simulink model "Lab5"  (R2017b)
settings: Solver=VariableStepAuto  StartTime=0.0  StopTime=200  RelTol=1e-3
libraries: cstblocks x8
settings Model: Creator=kelem  LastModifiedBy=kelem

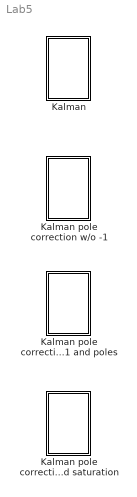
== system Lab5 ==
  Kalman : Subsystem
  Kalman pole correction w/o -1 : Subsystem
  Kalman pole correction1 w/o -1 and poles : Subsystem
  Kalman pole correction1 w/o -1 and poles and saturation : Subsystem

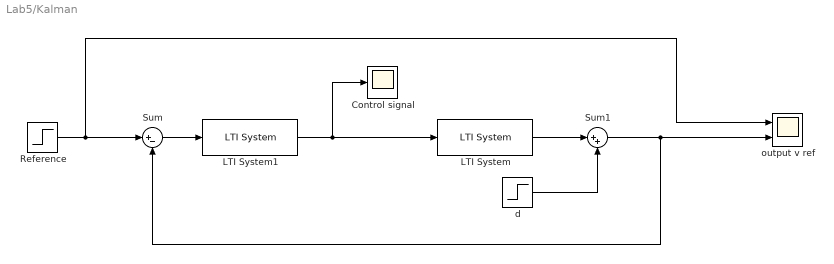
== system Lab5/Kalman ==
  "Control signal " : Scope
  LTI System : cstblocks/LTI System  sys=Hf  IC=[]
  LTI System1 : cstblocks/LTI System  sys=Hkc1  IC=[]
  Reference : Step  SampleTime=0
  Sum : Sum  Inputs=|+-
  Sum1 : Sum  Inputs=|++
  d : Step  SampleTime=50
  "output v ref " : Scope  NumInputPorts=2
  wires:
  LTI System1/1 -> LTI System/1, "Control signal "/1
  Sum/1 -> LTI System1/1
  d/1 -> Sum1/2
  Reference/1 -> Sum/1, "output v ref "/1
  Sum1/1 -> Sum/2, "output v ref "/2
  LTI System/1 -> Sum1/1

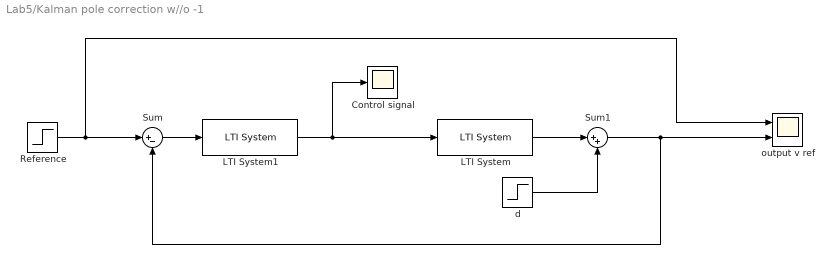
== system Lab5/Kalman pole correction w//o -1 ==
  "Control signal " : Scope
  LTI System : cstblocks/LTI System  sys=Hf  IC=[]
  LTI System1 : cstblocks/LTI System  sys=Hkc2  IC=[]
  Reference : Step  SampleTime=0
  Sum : Sum  Inputs=|+-
  Sum1 : Sum  Inputs=|++
  d : Step  SampleTime=50
  "output v ref " : Scope  NumInputPorts=2
  wires:
  LTI System1/1 -> LTI System/1, "Control signal "/1
  Sum/1 -> LTI System1/1
  d/1 -> Sum1/2
  Reference/1 -> Sum/1, "output v ref "/1
  Sum1/1 -> Sum/2, "output v ref "/2
  LTI System/1 -> Sum1/1

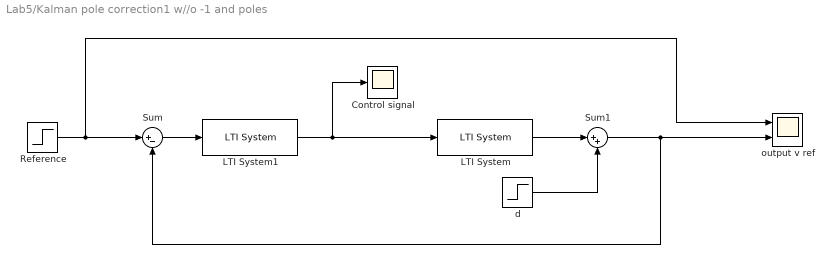
== system Lab5/Kalman pole correction1 w//o -1 and poles ==
  "Control signal " : Scope
  LTI System : cstblocks/LTI System  sys=Hf  IC=[]
  LTI System1 : cstblocks/LTI System  sys=Hkc3  IC=[]
  Reference : Step  SampleTime=0
  Sum : Sum  Inputs=|+-
  Sum1 : Sum  Inputs=|++
  d : Step  SampleTime=50
  "output v ref " : Scope  NumInputPorts=2
  wires:
  LTI System1/1 -> LTI System/1, "Control signal "/1
  Sum/1 -> LTI System1/1
  d/1 -> Sum1/2
  Reference/1 -> Sum/1, "output v ref "/1
  Sum1/1 -> Sum/2, "output v ref "/2
  LTI System/1 -> Sum1/1

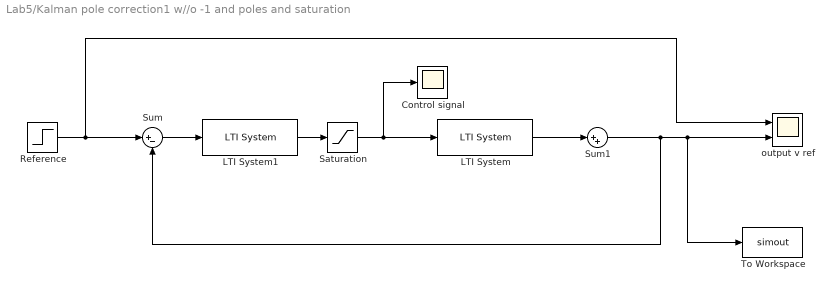
== system Lab5/Kalman pole correction1 w//o -1 and poles and saturation ==
  "Control signal " : Scope
  LTI System : cstblocks/LTI System  sys=Hf  IC=[]
  LTI System1 : cstblocks/LTI System  sys=Hkc3  IC=[]
  Reference : Step  SampleTime=0
  Saturation : Saturate
  Sum : Sum  Inputs=|+-
  Sum1 : Sum  Inputs=|++
  To Workspace : ToWorkspace  VariableName=simout  SaveFormat=Timeseries  SampleTime=-1
  "output v ref " : Scope  NumInputPorts=2
  wires:
  LTI System1/1 -> Saturation/1
  Sum/1 -> LTI System1/1
  Reference/1 -> Sum/1, "output v ref "/1
  Sum1/1 -> Sum/2, To Workspace/1, "output v ref "/2
  LTI System/1 -> Sum1/1
  Saturation/1 -> LTI System/1, "Control signal "/1
